simulink model "px4demo_attitude_system_GCS_combined_AttiGain3"  (R2016b)
settings: Solver=FixedStepDiscrete  StartTime=0.0  StopTime=inf  RelTol=1e-3
PostLoadFcn:
  | kFactor = 1.2;
  | 
  | KpRollAttitude = 0.630138625117681 / kFactor;
  | KiRollAttitude = 0.0552303199591522 / kFactor;
  | 
  | KpPitchAttitude = 0.630138625117681 / kFactor;
  | KiPitchAttitude = 0.0552303199591522 / kFactor;
  | 
  | KpRollRate = 1.31533836563383 / kFactor;
  | KiRollRate = 0.460338699849681 / kFactor;
  | 
  | KpPitchRate = 1.31533836563383 / kFactor;
  | KiPitchRate = 0.460338699849681 / kFactor;
  | 
  | KpYawRate = 1.31533836563383 / kFactor;
  | KiYawRate = 0.460338699849681 / kFactor;
undefined symbols (not defined in the file or in its folder): PX4_TUNE_ENUM, RGBLED_COLOR_ENUM, RGBLED_MODE_ENUM
libraries: pixhawk_slib_sensors_actuators x7, simulink x6, pixhawk_slib_ADC_serial x1
settings Model: Creator=Steve  LastModifiedBy=E6320
settings SolverCC: AutoInsertRateTranBlk=on
settings DataIOCC: LimitDataPoints=on  SaveFormat=Array
settings OptimizationCC: DefaultParameterBehavior=Inlined  LifeSpan=1  MaxStackSize=64
settings DebuggingCC: SolverPrmCheckMsg=warning  AllowSymbolicDim=off  SFUnexpectedBacktrackingDiag=warning  SFNoUnconditionalDefaultTransitionDiag=warning  SFExecutionAtInitializationDiag=none
settings HardwareCC: ProdBitPerPointer=32  ProdBitPerSizeT=32  ProdBitPerPtrDiffT=32  ProdLargestAtomicInteger=Long  ProdLargestAtomicFloat=Double  ProdWordSize=32  ProdHWDeviceType=ARM Compatible->ARM Cortex
settings ModelReferenceCC: PropagateSignalLabelsOutOfModel=off
settings RTWCC: SystemTargetFile=ert.tlc  HardwareBoard=Pixhawk PX4  TemplateMakefile=ert_default_tmf  Description=Embedded Coder  GenerateReport=on  Toolchain=Pixhawk Toolchain  IncludeHyperlinkInReport=on  LaunchReport=on  GenerateTraceReport=on  GenerateTraceReportSl=on  GenerateTraceReportSf=on  GenerateTraceReportEml=on  GenerateCodeMetricsReport=on
settings CodeAppCC: IgnoreCustomStorageClasses=off
settings ERTTargetCC: CodeReplacementLibrary=GCC ARM Cortex-A9  ExtModeTransport=1  ExtModeMexFile=ext_serial_win32_comm  ExtModeMexArgs=/dev/serial  ERTCustomFileTemplate=PX4_codertarget_file_process.tlc  ConvertIfToSwitch=off  SuppressUnreachableDefaultCases=off
settings ConfigComp: CovMetricSettings=dw  CovHtmlReporting=on  CovSaveCumulativeToWorkspaceVar=on  CovSaveSingleToWorkspaceVar=on  CovExternalEMLEnable=off  CovSFcnEnable=off

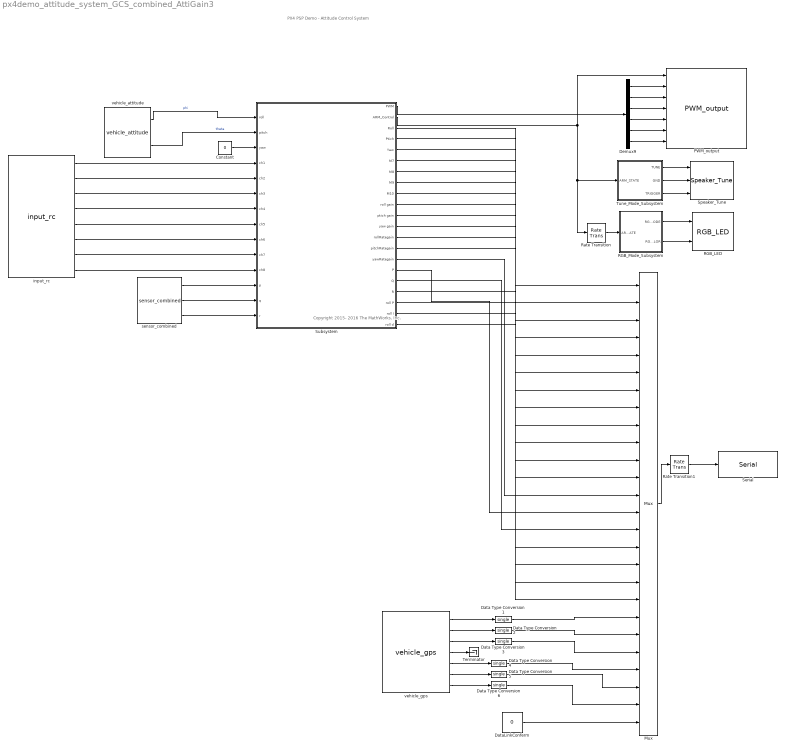
== system px4demo_attitude_system_GCS_combined_AttiGain3 ==
  note: PX4 PSP Demo - Attitude Control System
  note: Copyright 2015- 2016 The MathWorks, Inc.
  Constant : Constant  Value=0  OutDataTypeStr=single
  Data Type Conversion{1..6} (6 alike) : DataTypeConversion  OutDataTypeStr=single
  DataLinkConferm : Constant  Value=0  OutDataTypeStr=single
  Demux9 : Demux  Outputs=6
  Mux : Mux  Inputs=26
  PWM_output : pixhawk_slib_sensors_actuators/PWM_output  pwm_rate=250Hz  show_pwm1=on  show_pwm2=on  show_pwm3=on  show_pwm4=on  show_pwm5=on  show_pwm6=on  show_pwm7=off  show_pwm8=off
  RGB_LED : pixhawk_slib_sensors_actuators/RGB_LED
  RGB_Mode_Subsystem : Subsystem
  Rate Transition : RateTransition  OutPortSampleTime=1
  Rate Transition1 : RateTransition  OutPortSampleTime=1
  Serial : pixhawk_slib_ADC_serial/Serial  DeviceName=/dev/ttyS1  ReadOrWrite=Writing  BaudRateStr=57600  block=off  WriteStatus=on  Terminator=off  Header=off  NumBytesRead=4  TerminatorChar=\n  HeaderData=single('XD')  SimulateUsing=Code generation
  Speaker_Tune : pixhawk_slib_sensors_actuators/Speaker_Tune
  Subsystem : Subsystem
  Terminator : Terminator
  Tune_Mode_Subsystem : Subsystem
  input_rc : pixhawk_slib_sensors_actuators/input_rc  sampletime=1/250  channel1=on  channel2=on  channel3=on  channel4=on  channel5=on  channel6=on  channel7=on  channel8=on  ch_count=off  rssi=off  rc_failsafe=off  rc_lost=off  rc_inputsource=off
  sensor_combined : pixhawk_slib_sensors_actuators/sensor_combined  sampletime=1/250  show_mag=off  show_acc=off  show_gyro=on  show_baro=off  show_ts=off
  vehicle_attitude : pixhawk_slib_sensors_actuators/vehicle_attitude  sampletime=1/250  show_r=on  show_p=on  show_y=off  show_q=off
  vehicle_gps : pixhawk_slib_sensors_actuators/vehicle_gps  sampletime=1/250  show_ts_pos=off  show_alt=on  show_ts_gps=off  show_vel=on  show_fixtype=on  show_numsat=on
  wires:
  Demux9/6 -> PWM_output/7
  Demux9/5 -> PWM_output/6
  Demux9/4 -> PWM_output/5
  Demux9/2 -> PWM_output/3
  Demux9/3 -> PWM_output/4
  Demux9/1 -> PWM_output/2
  RGB_Mode_Subsystem/1(RGB_MODE) -> RGB_LED/1
  RGB_Mode_Subsystem/2(RGB_COLOR) -> RGB_LED/2
  Tune_Mode_Subsystem/1(TUNE) -> Speaker_Tune/1
  Tune_Mode_Subsystem/2(GND) -> Speaker_Tune/2
  Tune_Mode_Subsystem/3(TRIGGER) -> Speaker_Tune/3
  Subsystem/2(ARM_Control) -> PWM_output/1, Tune_Mode_Subsystem/1(ARM_STATE), Rate Transition/1
  vehicle_attitude/1 -> Subsystem/1(roll)  "phi"
  vehicle_attitude/2 -> Subsystem/2(pitch)  "theta"
  input_rc/1 -> Subsystem/4(ch1)
  input_rc/2 -> Subsystem/5(ch2)
  input_rc/3 -> Subsystem/6(ch3)
  input_rc/4 -> Subsystem/7(ch4)
  input_rc/5 -> Subsystem/8(ch5)
  Subsystem/1(PWM) -> Demux9/1
  Rate Transition/1 -> RGB_Mode_Subsystem/1(ARM_STATE)
  Mux/1 -> Rate Transition1/1
  Rate Transition1/1 -> Serial/1
  Subsystem/3(Roll) -> Mux/1
  Subsystem/4(Ptich) -> Mux/2
  Subsystem/5(Yaw) -> Mux/3
  Subsystem/6(M7) -> Mux/4
  Subsystem/7(M8) -> Mux/5
  Subsystem/8(M9) -> Mux/6
  Subsystem/9(M10) -> Mux/7
  Subsystem/10(roll gain) -> Mux/8
  Subsystem/11(ptich gain) -> Mux/9
  Subsystem/12(yaw gain) -> Mux/10
  Subsystem/13(rollRategain) -> Mux/11
  Subsystem/14(pitchRategain) -> Mux/12
  Subsystem/15(yawRategain) -> Mux/13
  sensor_combined/1 -> Subsystem/12(p)
  sensor_combined/2 -> Subsystem/13(q)
  sensor_combined/3 -> Subsystem/14(r)
  Constant/1 -> Subsystem/3(yaw)
  input_rc/6 -> Subsystem/9(ch6)
  input_rc/7 -> Subsystem/10(ch7)
  input_rc/8 -> Subsystem/11(ch8)
  vehicle_gps/2 -> Data Type Conversion2/1
  vehicle_gps/1 -> Data Type Conversion1/1
  vehicle_gps/3 -> Data Type Conversion3/1
  vehicle_gps/5 -> Data Type Conversion4/1
  vehicle_gps/6 -> Data Type Conversion5/1
  vehicle_gps/7 -> Data Type Conversion6/1
  vehicle_gps/4 -> Terminator/1
  Data Type Conversion1/1 -> Mux/20
  Data Type Conversion2/1 -> Mux/21
  Data Type Conversion3/1 -> Mux/22
  Data Type Conversion4/1 -> Mux/23
  Data Type Conversion5/1 -> Mux/24
  Data Type Conversion6/1 -> Mux/25
  DataLinkConferm/1 -> Mux/26
  Subsystem/18(R) -> Mux/16
  Subsystem/17(Q) -> Mux/15
  Subsystem/16(P) -> Mux/14
  Subsystem/19(roll P) -> Mux/17
  Subsystem/20(roll I) -> Mux/18
  Subsystem/21(roll d) -> Mux/19

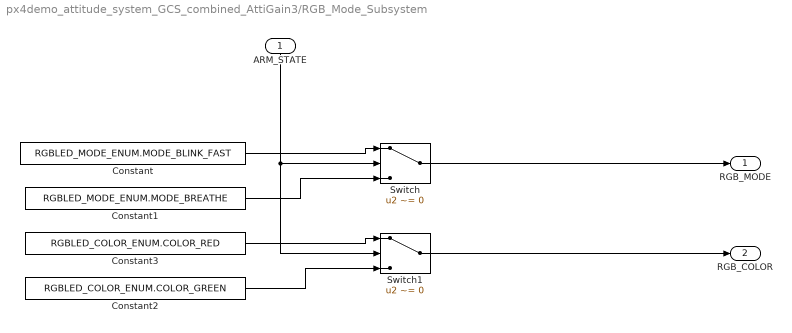
== system px4demo_attitude_system_GCS_combined_AttiGain3/RGB_Mode_Subsystem ==
  ARM_STATE : Inport
  Constant : Constant  Value=RGBLED_MODE_ENUM.MODE_BLINK_FAST  OutDataTypeStr=Enum: RGBLED_MODE_ENUM
  Constant1 : Constant  Value=RGBLED_MODE_ENUM.MODE_BREATHE  OutDataTypeStr=Enum: RGBLED_MODE_ENUM
  Constant2 : Constant  Value=RGBLED_COLOR_ENUM.COLOR_GREEN  OutDataTypeStr=Enum: RGBLED_COLOR_ENUM
  Constant3 : Constant  Value=RGBLED_COLOR_ENUM.COLOR_RED  OutDataTypeStr=Enum: RGBLED_COLOR_ENUM
  Switch : Switch  Criteria=u2 ~= 0  Threshold=1500  SampleTime=1/2
  Switch1 : Switch  Criteria=u2 ~= 0  Threshold=1500  SampleTime=1/2
  RGB_MODE : Outport
  RGB_COLOR : Outport  Port=2
  wires:
  ARM_STATE/1 -> Switch1/2, Switch/2
  Constant/1 -> Switch/1
  Constant1/1 -> Switch/3
  Switch/1 -> RGB_MODE/1
  Constant3/1 -> Switch1/1
  Constant2/1 -> Switch1/3
  Switch1/1 -> RGB_COLOR/1

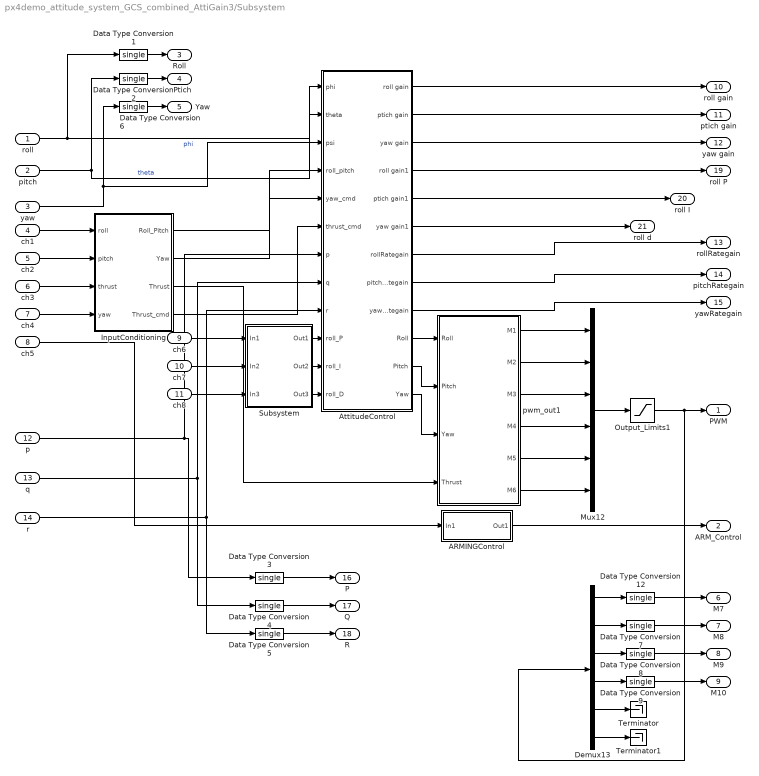
== system px4demo_attitude_system_GCS_combined_AttiGain3/Subsystem ==
  roll : Inport  OutDataTypeStr=single  PortDimensions=1
  pitch : Inport  Port=2  PortDimensions=1
  yaw : Inport  Port=3  PortDimensions=1
  ch1 : Inport  Port=4  OutDataTypeStr=uint16  PortDimensions=1
  ch2 : Inport  Port=5  OutDataTypeStr=uint16  PortDimensions=1
  ch3 : Inport  Port=6  OutDataTypeStr=uint16  PortDimensions=1
  ch4 : Inport  Port=7  OutDataTypeStr=uint16  PortDimensions=1
  ch5 : Inport  Port=8  OutDataTypeStr=uint16  PortDimensions=1  Interpolate=off
  ch6 : Inport  Port=9  OutDataTypeStr=uint16  PortDimensions=1
  ch7 : Inport  Port=10  OutDataTypeStr=uint16  PortDimensions=1
  ch8 : Inport  Port=11  OutDataTypeStr=uint16  PortDimensions=1
  p : Inport  Port=12  OutDataTypeStr=single  PortDimensions=1
  q : Inport  Port=13  OutDataTypeStr=single  PortDimensions=1
  r : Inport  Port=14  PortDimensions=1
  ARMINGControl : Subsystem
  AttitudeControl : Subsystem
  Data Type Conversion{1..9,12} (10 alike) : DataTypeConversion  OutDataTypeStr=single
  Demux13 : Demux  Outputs=6
  InputConditioning : Subsystem
  Mux12 : Mux  Inputs=6
  Output_Limits1 : Saturate  UpperLimit=2000  LowerLimit=1000
  Subsystem : Subsystem
  Terminator : Terminator
  Terminator1 : Terminator
  pwm_out1 : MATLAB Function  TreatAsAtomicUnit=on  SystemSampleTime=0.004
  PWM : Outport  PortDimensions=6
  ARM_Control : Outport  Port=2  PortDimensions=1
  Roll : Outport  Port=3  PortDimensions=1
  Ptich : Outport  Port=4  PortDimensions=1
  Yaw : Outport  Port=5  PortDimensions=1
  M7 : Outport  Port=6  PortDimensions=1
  M8 : Outport  Port=7  PortDimensions=1
  M9 : Outport  Port=8  PortDimensions=1
  M10 : Outport  Port=9  PortDimensions=1
  roll gain : Outport  Port=10
  ptich gain : Outport  Port=11
  yaw gain : Outport  Port=12
  rollRategain : Outport  Port=13
  pitchRategain : Outport  Port=14
  yawRategain : Outport  Port=15
  P : Outport  Port=16  PortDimensions=1
  Q : Outport  Port=17  PortDimensions=1
  R : Outport  Port=18  PortDimensions=1
  roll P : Outport  Port=19
  roll I : Outport  Port=20
  roll d : Outport  Port=21
  wires:
  Mux12/1 -> Output_Limits1/1
  InputConditioning/3(Thrust) -> pwm_out1/4(Thrust)
  roll/1 -> Data Type Conversion1/1, AttitudeControl/1(phi)  "phi"
  pitch/1 -> AttitudeControl/2(theta), Data Type Conversion2/1  "theta"
  InputConditioning/1(Roll_Pitch) -> AttitudeControl/4(roll_pitch)
  InputConditioning/2(Yaw) -> AttitudeControl/5(yaw_cmd)
  p/1 -> Data Type Conversion3/1, AttitudeControl/7(p)
  q/1 -> AttitudeControl/8(q), Data Type Conversion4/1
  r/1 -> AttitudeControl/9(r), Data Type Conversion5/1
  AttitudeControl/10(Roll) -> pwm_out1/1(Roll)
  AttitudeControl/11(Pitch) -> pwm_out1/2(Pitch)
  AttitudeControl/12(Yaw) -> pwm_out1/3(Yaw)
  ch5/1 -> ARMINGControl/1(In1)
  pwm_out1/1(M1) -> Mux12/1
  pwm_out1/2(M2) -> Mux12/2
  pwm_out1/3(M3) -> Mux12/3
  pwm_out1/4(M4) -> Mux12/4
  pwm_out1/5(M5) -> Mux12/5
  pwm_out1/6(M6) -> Mux12/6
  ch1/1 -> InputConditioning/1(roll)
  ch2/1 -> InputConditioning/2(pitch)
  ch4/1 -> InputConditioning/4(yaw)
  ch3/1 -> InputConditioning/3(thrust)
  ARMINGControl/1(Out1) -> ARM_Control/1
  InputConditioning/4(Thrust_cmd) -> AttitudeControl/6(thrust_cmd)
  Data Type Conversion1/1 -> Roll/1
  Data Type Conversion2/1 -> Ptich/1
  Output_Limits1/1 -> Demux13/1, PWM/1
  Data Type Conversion12/1 -> M7/1
  Data Type Conversion7/1 -> M8/1
  Data Type Conversion8/1 -> M9/1
  Data Type Conversion9/1 -> M10/1
  Demux13/1 -> Data Type Conversion12/1
  Demux13/2 -> Data Type Conversion7/1
  Demux13/3 -> Data Type Conversion8/1
  Demux13/4 -> Data Type Conversion9/1
  Demux13/5 -> Terminator/1
  AttitudeControl/1(roll gain) -> roll gain/1
  AttitudeControl/2(ptich gain) -> ptich gain/1
  AttitudeControl/7(rollRategain) -> rollRategain/1
  AttitudeControl/8(pitchRategain) -> pitchRategain/1
  Demux13/6 -> Terminator1/1
  Data Type Conversion3/1 -> P/1
  Data Type Conversion4/1 -> Q/1
  Data Type Conversion5/1 -> R/1
  AttitudeControl/9(yawRategain) -> yawRategain/1
  yaw/1 -> AttitudeControl/3(psi), Data Type Conversion6/1
  Data Type Conversion6/1 -> Yaw/1
  AttitudeControl/3(yaw gain) -> yaw gain/1
  AttitudeControl/6(yaw gain1) -> roll d/1
  AttitudeControl/5(ptich gain1) -> roll I/1
  AttitudeControl/4(roll gain1) -> roll P/1
  ch6/1 -> Subsystem/1(In1)
  ch7/1 -> Subsystem/2(In2)
  ch8/1 -> Subsystem/3(In3)
  Subsystem/1(Out1) -> AttitudeControl/10(roll_P)
  Subsystem/3(Out3) -> AttitudeControl/12(roll_D)
  Subsystem/2(Out2) -> AttitudeControl/11(roll_I)

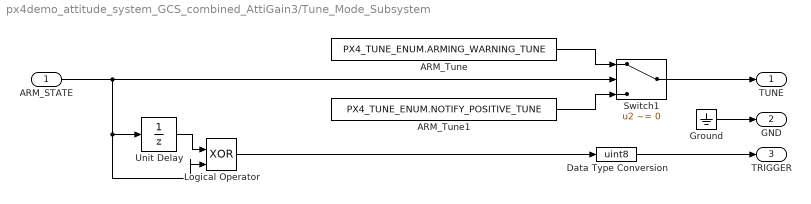
== system px4demo_attitude_system_GCS_combined_AttiGain3/Tune_Mode_Subsystem ==
  ARM_STATE : Inport
  ARM_Tune : Constant  Value=PX4_TUNE_ENUM.ARMING_WARNING_TUNE  OutDataTypeStr=Enum: PX4_TUNE_ENUM
  ARM_Tune1 : Constant  Value=PX4_TUNE_ENUM.NOTIFY_POSITIVE_TUNE  OutDataTypeStr=Enum: PX4_TUNE_ENUM
  Data Type Conversion : DataTypeConversion  OutDataTypeStr=uint8
  Ground : Ground
  Logical Operator : Logic  Operator=XOR  IconShape=distinctive  AllPortsSameDT=off  OutDataTypeStr=boolean
  Switch1 : Switch  Criteria=u2 ~= 0  Threshold=1500
  Unit Delay : UnitDelay  SampleTime=-1
  TUNE : Outport
  GND : Outport  Port=2
  TRIGGER : Outport  Port=3
  wires:
  Ground/1 -> GND/1
  Data Type Conversion/1 -> TRIGGER/1
  Switch1/1 -> TUNE/1
  ARM_Tune/1 -> Switch1/1
  ARM_Tune1/1 -> Switch1/3
  ARM_STATE/1 -> Logical Operator/2, Unit Delay/1, Switch1/2
  Unit Delay/1 -> Logical Operator/1
  Logical Operator/1 -> Data Type Conversion/1

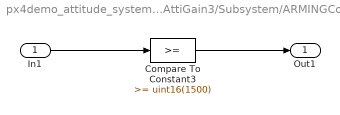
== system px4demo_attitude_system_GCS_combined_AttiGain3/Subsystem/ARMINGControl ==
  In1 : Inport
  Compare To Constant3 : simulink/Logic and Bit Operations/Compare To Constant  relop=>=  const=uint16(1500)  OutDataTypeStr=boolean
  Out1 : Outport
  wires:
  Compare To Constant3/1 -> Out1/1
  In1/1 -> Compare To Constant3/1

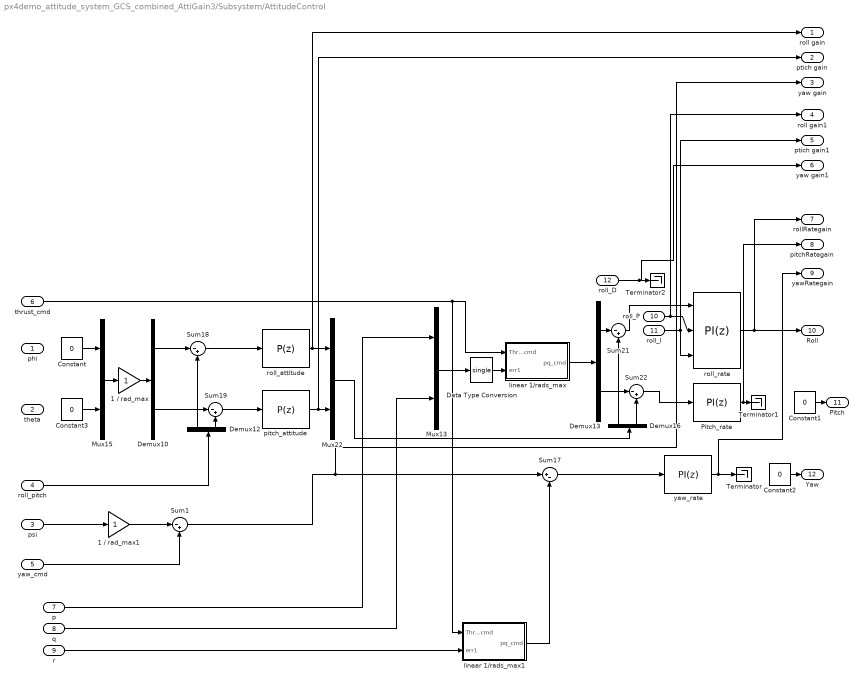
== system px4demo_attitude_system_GCS_combined_AttiGain3/Subsystem/AttitudeControl ==
  phi : Inport
  theta : Inport  Port=2
  psi : Inport  Port=3
  roll_pitch : Inport  Port=4
  yaw_cmd : Inport  Port=5
  thrust_cmd : Inport  Port=6
  p : Inport  Port=7
  q : Inport  Port=8
  r : Inport  Port=9
  roll_P : Inport  Port=10
  roll_I : Inport  Port=11
  roll_D : Inport  Port=12
  1 / rad_max : Gain
  1 / rad_max1 : Gain
  Constant{,1..3} (4 alike) : Constant  Value=0  OutDataTypeStr=single
  Data Type Conversion : DataTypeConversion  OutDataTypeStr=single
  Demux{10,12..13,16} (4 alike) : Demux  Outputs=2
  Mux13 : Mux  Inputs=2
  Mux15 : Mux  Inputs=2
  Mux22 : Mux  Inputs=2
  Pitch_rate : simulink/Continuous/PID Controller  Controller=PI  TimeDomain=Discrete-time  SampleTime=-1  IntegratorMethod=Forward Euler  FilterMethod=Forward Euler  Form=Parallel  UseFilter=on  ControllerParametersSource=internal  P=5  I=0.01  D=0.0024  N=100  InitialConditionSource=internal  InitialConditionForIntegrator=0  InitialConditionForFilter=0  ExternalReset=none  LimitOutput=on  UpperSaturationLimit=1  LowerSaturationLimit=-1  LinearizeAsGain=on  AntiWindupMode=clamping  Kb=1  TrackingMode=off  Kt=1  PParamMin=[]  PParamMax=[]  IParamMin=[]  IParamMax=[]  DParamMin=[]  DParamMax=[]  NParamMin=[]  NParamMax=[]  KbParamMin=[]  KbParamMax=[]  KtParamMin=[]  KtParamMax=[]  POutMin=[]  POutMax=[]  IOutMin=[]  IOutMax=[]  DOutMin=[]  DOutMax=[]  NOutMin=[]  NOutMax=[]  KbOutMin=[]  KbOutMax=[]  KtOutMin=[]  KtOutMax=[]  IntegratorOutMin=[]  IntegratorOutMax=[]  FilterOutMin=[]  FilterOutMax=[]  SumOutMin=[]  SumOutMax=[]  SumI1OutMin=[]  SumI1OutMax=[]  SumI2OutMin=[]  SumI2OutMax=[]  SumI3OutMin=[]  SumI3OutMax=[]  SumDOutMin=[]  SumDOutMax=[]  SaturationOutMin=[]  SaturationOutMax=[]  IntegratorContinuousStateAttributes=''  IntegratorStateMustResolveToSignalObject=off  IntegratorRTWStateStorageClass=Auto  FilterContinuousStateAttributes=''  FilterStateMustResolveToSignalObject=off  FilterRTWStateStorageClass=Auto  DifferentiatorICPrevScaledInput=0  DifferentiatorOutMin=[]  DifferentiatorOutMax=[]
  Sum{1,18..19,21..22} (5 alike) : Sum  Inputs=|-+
  Sum17 : Sum  Inputs=|+-
  Terminator : Terminator
  Terminator1 : Terminator
  Terminator2 : Terminator
  linear 1/rads_max : MATLAB Function  TreatAsAtomicUnit=on
  linear 1/rads_max1 : MATLAB Function  TreatAsAtomicUnit=on
  pitch_attitude : simulink/Continuous/PID Controller  Controller=P  TimeDomain=Discrete-time  SampleTime=-1  IntegratorMethod=Forward Euler  FilterMethod=Forward Euler  Form=Parallel  UseFilter=on  ControllerParametersSource=internal  P=1  I=0.05  D=0.01  N=100  InitialConditionSource=internal  InitialConditionForIntegrator=0  InitialConditionForFilter=0  ExternalReset=none  LimitOutput=on  UpperSaturationLimit=1  LowerSaturationLimit=-1  LinearizeAsGain=on  AntiWindupMode=clamping  Kb=1  TrackingMode=off  Kt=1  PParamMin=[]  PParamMax=[]  IParamMin=[]  IParamMax=[]  DParamMin=[]  DParamMax=[]  NParamMin=[]  NParamMax=[]  KbParamMin=[]  KbParamMax=[]  KtParamMin=[]  KtParamMax=[]  POutMin=[]  POutMax=[]  IOutMin=[]  IOutMax=[]  DOutMin=[]  DOutMax=[]  NOutMin=[]  NOutMax=[]  KbOutMin=[]  KbOutMax=[]  KtOutMin=[]  KtOutMax=[]  IntegratorOutMin=[]  IntegratorOutMax=[]  FilterOutMin=[]  FilterOutMax=[]  SumOutMin=[]  SumOutMax=[]  SumI1OutMin=[]  SumI1OutMax=[]  SumI2OutMin=[]  SumI2OutMax=[]  SumI3OutMin=[]  SumI3OutMax=[]  SumDOutMin=[]  SumDOutMax=[]  SaturationOutMin=[]  SaturationOutMax=[]  IntegratorContinuousStateAttributes=''  IntegratorStateMustResolveToSignalObject=off  IntegratorRTWStateStorageClass=Auto  FilterContinuousStateAttributes=''  FilterStateMustResolveToSignalObject=off  FilterRTWStateStorageClass=Auto  DifferentiatorICPrevScaledInput=0  DifferentiatorOutMin=[]  DifferentiatorOutMax=[]
  roll_attitude : simulink/Continuous/PID Controller  Controller=P  TimeDomain=Discrete-time  SampleTime=-1  IntegratorMethod=Forward Euler  FilterMethod=Forward Euler  Form=Parallel  UseFilter=on  ControllerParametersSource=internal  P=1  I=0.04  D=0.01  N=100  InitialConditionSource=internal  InitialConditionForIntegrator=0  InitialConditionForFilter=0  ExternalReset=none  LimitOutput=on  UpperSaturationLimit=1  LowerSaturationLimit=-1  LinearizeAsGain=on  AntiWindupMode=clamping  Kb=1  TrackingMode=off  Kt=1  PParamMin=[]  PParamMax=[]  IParamMin=[]  IParamMax=[]  DParamMin=[]  DParamMax=[]  NParamMin=[]  NParamMax=[]  KbParamMin=[]  KbParamMax=[]  KtParamMin=[]  KtParamMax=[]  POutMin=[]  POutMax=[]  IOutMin=[]  IOutMax=[]  DOutMin=[]  DOutMax=[]  NOutMin=[]  NOutMax=[]  KbOutMin=[]  KbOutMax=[]  KtOutMin=[]  KtOutMax=[]  IntegratorOutMin=[]  IntegratorOutMax=[]  FilterOutMin=[]  FilterOutMax=[]  SumOutMin=[]  SumOutMax=[]  SumI1OutMin=[]  SumI1OutMax=[]  SumI2OutMin=[]  SumI2OutMax=[]  SumI3OutMin=[]  SumI3OutMax=[]  SumDOutMin=[]  SumDOutMax=[]  SaturationOutMin=[]  SaturationOutMax=[]  IntegratorContinuousStateAttributes=''  IntegratorStateMustResolveToSignalObject=off  IntegratorRTWStateStorageClass=Auto  FilterContinuousStateAttributes=''  FilterStateMustResolveToSignalObject=off  FilterRTWStateStorageClass=Auto  DifferentiatorICPrevScaledInput=0  DifferentiatorOutMin=[]  DifferentiatorOutMax=[]
  roll_rate : simulink/Continuous/PID Controller  Controller=PI  TimeDomain=Discrete-time  SampleTime=-1  IntegratorMethod=Forward Euler  FilterMethod=Forward Euler  Form=Parallel  UseFilter=on  ControllerParametersSource=external  P=5  I=0.01  D=0.015  N=100  InitialConditionSource=internal  InitialConditionForIntegrator=0  InitialConditionForFilter=0  ExternalReset=none  LimitOutput=on  UpperSaturationLimit=1  LowerSaturationLimit=-1  LinearizeAsGain=on  AntiWindupMode=clamping  Kb=1  TrackingMode=off  Kt=1  PParamMin=[]  PParamMax=[]  IParamMin=[]  IParamMax=[]  DParamMin=[]  DParamMax=[]  NParamMin=[]  NParamMax=[]  KbParamMin=[]  KbParamMax=[]  KtParamMin=[]  KtParamMax=[]  POutMin=[]  POutMax=[]  IOutMin=[]  IOutMax=[]  DOutMin=[]  DOutMax=[]  NOutMin=[]  NOutMax=[]  KbOutMin=[]  KbOutMax=[]  KtOutMin=[]  KtOutMax=[]  IntegratorOutMin=[]  IntegratorOutMax=[]  FilterOutMin=[]  FilterOutMax=[]  SumOutMin=[]  SumOutMax=[]  SumI1OutMin=[]  SumI1OutMax=[]  SumI2OutMin=[]  SumI2OutMax=[]  SumI3OutMin=[]  SumI3OutMax=[]  SumDOutMin=[]  SumDOutMax=[]  SaturationOutMin=[]  SaturationOutMax=[]  IntegratorContinuousStateAttributes=''  IntegratorStateMustResolveToSignalObject=off  IntegratorRTWStateStorageClass=Auto  FilterContinuousStateAttributes=''  FilterStateMustResolveToSignalObject=off  FilterRTWStateStorageClass=Auto  DifferentiatorICPrevScaledInput=0  DifferentiatorOutMin=[]  DifferentiatorOutMax=[]
  yaw_rate : simulink/Continuous/PID Controller  Controller=PI  TimeDomain=Discrete-time  SampleTime=-1  IntegratorMethod=Forward Euler  FilterMethod=Forward Euler  Form=Parallel  UseFilter=on  ControllerParametersSource=internal  P=0.87  I=0.3  D=0  N=100  InitialConditionSource=internal  InitialConditionForIntegrator=0  InitialConditionForFilter=0  ExternalReset=none  LimitOutput=on  UpperSaturationLimit=1  LowerSaturationLimit=-1  LinearizeAsGain=on  AntiWindupMode=back-calculation  Kb=1  TrackingMode=off  Kt=1  PParamMin=[]  PParamMax=[]  IParamMin=[]  IParamMax=[]  DParamMin=[]  DParamMax=[]  NParamMin=[]  NParamMax=[]  KbParamMin=[]  KbParamMax=[]  KtParamMin=[]  KtParamMax=[]  POutMin=[]  POutMax=[]  IOutMin=[]  IOutMax=[]  DOutMin=[]  DOutMax=[]  NOutMin=[]  NOutMax=[]  KbOutMin=[]  KbOutMax=[]  KtOutMin=[]  KtOutMax=[]  IntegratorOutMin=[]  IntegratorOutMax=[]  FilterOutMin=[]  FilterOutMax=[]  SumOutMin=[]  SumOutMax=[]  SumI1OutMin=[]  SumI1OutMax=[]  SumI2OutMin=[]  SumI2OutMax=[]  SumI3OutMin=[]  SumI3OutMax=[]  SumDOutMin=[]  SumDOutMax=[]  SaturationOutMin=[]  SaturationOutMax=[]  IntegratorContinuousStateAttributes=''  IntegratorStateMustResolveToSignalObject=off  IntegratorRTWStateStorageClass=Auto  FilterContinuousStateAttributes=''  FilterStateMustResolveToSignalObject=off  FilterRTWStateStorageClass=Auto  DifferentiatorICPrevScaledInput=0  DifferentiatorOutMin=[]  DifferentiatorOutMax=[]
  roll gain : Outport
  ptich gain : Outport  Port=2
  yaw gain : Outport  Port=3
  roll gain1 : Outport  Port=4
  ptich gain1 : Outport  Port=5
  yaw gain1 : Outport  Port=6
  rollRategain : Outport  Port=7
  pitchRategain : Outport  Port=8
  yawRategain : Outport  Port=9
  Roll : Outport  Port=10
  Pitch : Outport  Port=11
  Yaw : Outport  Port=12
  wires:
  Mux22/1 -> Demux16/1
  Mux15/1 -> 1 / rad_max/1
  roll_rate/1 -> rollRategain/1, Roll/1
  Sum19/1 -> pitch_attitude/1
  pitch_attitude/1 -> Mux22/2, ptich gain/1
  Demux16/1 -> Sum21/2
  roll_pitch/1 -> Demux12/1
  Demux16/2 -> Sum22/2
  Demux12/1 -> Sum18/2
  Demux12/2 -> Sum19/2
  Demux10/1 -> Sum18/1
  Demux10/2 -> Sum19/1
  1 / rad_max/1 -> Demux10/1
  Sum18/1 -> roll_attitude/1
  Sum22/1 -> Pitch_rate/1
  Sum17/1 -> yaw_rate/1
  Demux13/1 -> Sum21/1
  Demux13/2 -> Sum22/1
  Sum21/1 -> roll_rate/1
  Data Type Conversion/1 -> linear 1/rads_max/2(err1)
  Mux13/1 -> Data Type Conversion/1
  linear 1/rads_max/1(pq_cmd) -> Demux13/1
  thrust_cmd/1 -> linear 1/rads_max1/1(Thrust_cmd), linear 1/rads_max/1(Thrust_cmd)
  roll_attitude/1 -> roll gain/1, Mux22/1
  psi/1 -> 1 / rad_max1/1
  1 / rad_max1/1 -> Sum1/1
  yaw_cmd/1 -> Sum1/2
  linear 1/rads_max1/1(pq_cmd) -> Sum17/2
  Sum1/1 -> yaw gain/1, Sum17/1
  p/1 -> Mux13/1
  q/1 -> Mux13/2
  r/1 -> linear 1/rads_max1/2(err1)
  roll_P/1 -> roll gain1/1, roll_rate/2
  roll_I/1 -> ptich gain1/1, roll_rate/3
  roll_D/1 -> yaw gain1/1, Terminator2/1
  yaw_rate/1 -> Terminator/1, yawRategain/1
  Constant1/1 -> Pitch/1
  Pitch_rate/1 -> pitchRategain/1, Terminator1/1
  Constant2/1 -> Yaw/1
  Constant/1 -> Mux15/1
  Constant3/1 -> Mux15/2

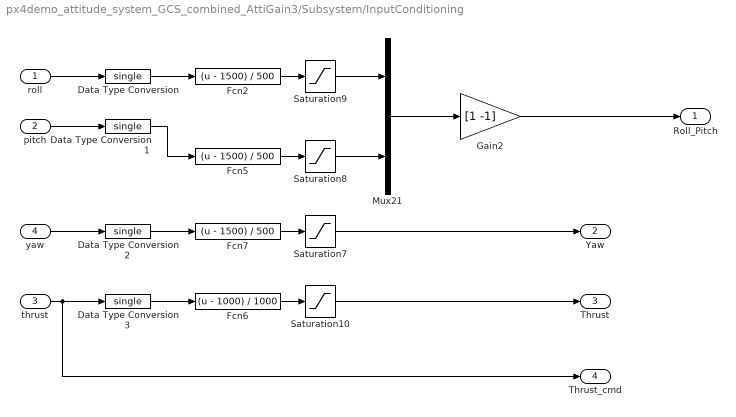
== system px4demo_attitude_system_GCS_combined_AttiGain3/Subsystem/InputConditioning ==
  roll : Inport
  pitch : Inport  Port=2
  thrust : Inport  Port=3
  yaw : Inport  Port=4
  Data Type Conversion{,1..3} (4 alike) : DataTypeConversion  OutDataTypeStr=single
  Fcn2 : Fcn  Expr=(u - 1500) / 500
  Fcn5 : Fcn  Expr=(u - 1500) / 500
  Fcn6 : Fcn  Expr=(u - 1000) / 1000
  Fcn7 : Fcn  Expr=(u - 1500) / 500
  Gain2 : Gain  Gain=[1 -1]  OutDataTypeStr=Inherit: Inherit via back propagation
  Mux21 : Mux  Inputs=2
  Saturation10 : Saturate  UpperLimit=1  LowerLimit=0
  Saturation7 : Saturate  UpperLimit=1  LowerLimit=-1
  Saturation8 : Saturate  UpperLimit=1  LowerLimit=-1
  Saturation9 : Saturate  UpperLimit=1  LowerLimit=-1
  Roll_Pitch : Outport
  Yaw : Outport  Port=2
  Thrust : Outport  Port=3
  Thrust_cmd : Outport  Port=4
  wires:
  Saturation10/1 -> Thrust/1
  Saturation7/1 -> Yaw/1
  Gain2/1 -> Roll_Pitch/1
  Mux21/1 -> Gain2/1
  Saturation8/1 -> Mux21/2
  Fcn6/1 -> Saturation10/1
  thrust/1 -> Thrust_cmd/1, Data Type Conversion3/1
  Fcn2/1 -> Saturation9/1
  Fcn5/1 -> Saturation8/1
  Saturation9/1 -> Mux21/1
  Fcn7/1 -> Saturation7/1
  yaw/1 -> Data Type Conversion2/1
  pitch/1 -> Data Type Conversion1/1
  roll/1 -> Data Type Conversion/1
  Data Type Conversion/1 -> Fcn2/1
  Data Type Conversion1/1 -> Fcn5/1
  Data Type Conversion2/1 -> Fcn7/1
  Data Type Conversion3/1 -> Fcn6/1

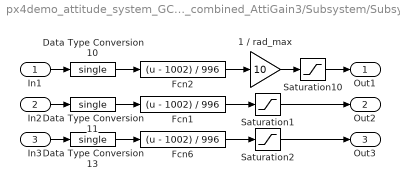
== system px4demo_attitude_system_GCS_combined_AttiGain3/Subsystem/Subsystem ==
  In1 : Inport
  In2 : Inport  Port=2
  In3 : Inport  Port=3
  1 / rad_max : Gain  Gain=10
  Data Type Conversion10 : DataTypeConversion  OutDataTypeStr=single
  Data Type Conversion11 : DataTypeConversion  OutDataTypeStr=single
  Data Type Conversion13 : DataTypeConversion  OutDataTypeStr=single
  Fcn1 : Fcn  Expr=(u - 1002) / 996
  Fcn2 : Fcn  Expr=(u - 1002) / 996
  Fcn6 : Fcn  Expr=(u - 1002) / 996
  Saturation1 : Saturate  UpperLimit=1  LowerLimit=0
  Saturation10 : Saturate  UpperLimit=3  LowerLimit=0
  Saturation2 : Saturate  UpperLimit=1  LowerLimit=0
  Out1 : Outport
  Out2 : Outport  Port=2
  Out3 : Outport  Port=3
  wires:
  Data Type Conversion13/1 -> Fcn6/1
  Fcn6/1 -> Saturation2/1
  Fcn2/1 -> 1 / rad_max/1
  Data Type Conversion11/1 -> Fcn1/1
  In3/1 -> Data Type Conversion13/1
  Data Type Conversion10/1 -> Fcn2/1
  In2/1 -> Data Type Conversion11/1
  In1/1 -> Data Type Conversion10/1
  Fcn1/1 -> Saturation1/1
  Saturation10/1 -> Out1/1
  Saturation1/1 -> Out2/1
  Saturation2/1 -> Out3/1
  1 / rad_max/1 -> Saturation10/1

== matlab function px4demo_attitude_system_GCS_combined_AttiGain3/Subsystem/AttitudeControl/linear 1//rads_max1 ==
  data: Thrust_cmd input; pq_cmd output; err1 input
function pq_cmd  = fcn(Thrust_cmd,err1)

% T = 1225. rads max = 3
% T = 1400. rads max = 20

T1 = 1225; T2 = 1400;
p1 = 4; p2 = 25;
m = (p2-p1)/(T2-T1);
b = p1 - m*T1;

y = single(max(4,m*min(1946,max(1135,Thrust_cmd)) + b));

pq_cmd = single(err1/y);

== matlab function px4demo_attitude_system_GCS_combined_AttiGain3/Subsystem/AttitudeControl/linear 1//rads_max ==
  data: Thrust_cmd input; pq_cmd output; err1 input
function pq_cmd  = fcn(Thrust_cmd,err1)

% T = 1225. rads max = 3
% T = 1400. rads max = 20

T1 = 1225; T2 = 1400;
p1 = 3; p2 = 12;
m = (p2-p1)/(T2-T1);
b = p1 - m*T1;

y = single(max(3,m*min(1946,max(1135,Thrust_cmd)) + b));

pq_cmd = single(err1/y);

== matlab function px4demo_attitude_system_GCS_combined_AttiGain3/Subsystem/pwm_out1 ==
  data: Roll input; M1 output; Pitch input; Yaw input; Thrust input; M2 output; M3 output; M4 output; M5 output; M6 output
function [M1, M2, M3, M4, M5, M6] = motor_mixer(Roll, Pitch, Yaw, Thrust)

idle_PWM = uint16(1145);

% Quad X
M1 = uint16(single(((Roll + Pitch - Yaw) / 2 * Thrust + Thrust) * single(1000))) + idle_PWM;
M2 = uint16(single(((-Roll + Pitch + Yaw) / 2 * Thrust + Thrust) * single(1000))) + idle_PWM;
M3 = uint16(single(((-Roll - Pitch - Yaw) / 2 * Thrust + Thrust) * single(1000))) + idle_PWM;
M4 = uint16(single(((Roll - Pitch + Yaw) / 2 * Thrust + Thrust) * single(1000))) + idle_PWM;
M5 = uint16(1000);
M6 = uint16(1000);
% M1 = uint16(single(((Roll + Pitch - Yaw)  + Thrust) * single(1000))) + idle_PWM;
% M2 = uint16(single(((-Roll + Pitch + Yaw)  + Thrust) * single(1000))) + idle_PWM;
% M3 = uint16(single(((-Roll - Pitch - Yaw)  + Thrust) * single(1000))) + idle_PWM;
% M4 = uint16(single(((Roll - Pitch + Yaw)  + Thrust) * single(1000))) + idle_PWM;
% M5 = uint16(1000);
% M6 = uint16(1000);

% Quad +
% M1 = ((Pitch - Yaw) * Thrust / 2 + Thrust) * 1000 + idle_PWM;
% M2 = ((-Roll + Yaw) * Thrust / 2 + Thrust) * 1000 + idle_PWM;
% M3 = ((-Pitch - Yaw) * Thrust / 2 + Thrust) * 1000 + idle_PWM;
% M4 = ((Roll + Yaw) * Thrust / 2 + Thrust) * 1000 + idle_PWM;
% M5 = 1000;
% M6 = 1000;
% M7 = 1000;
% M8 = 1000;

% Hex X
% M1 = ((Pitch + Roll / 2 - Yaw) * Thrust / 2 + Thrust) * 1000 + idle_PWM;
% M2 = ((Pitch - Roll / 2 + Yaw) * Thrust / 2 + Thrust) * 1000 + idle_PWM;
% M3 = ((-Roll - Yaw) * Thrust / 2 + Thrust) * 1000 + idle_PWM;
% M4 = ((-Pitch - Roll / 2 + Yaw) * Thrust / 2 + Thrust) * 1000 + idle_PWM;
% M5 = ((-Pitch + Roll / 2 - Yaw) * Thrust / 2 + Thrust) * 1000 + idle_PWM;
% M6 = ((Roll + Yaw) * Thrust / 2 + Thrust) * 1000 + idle_PWM;
% M7 = 1000;
% M8 = 1000;

% Hex X (From Adam)
% M1 = uint16(single(((-Roll - Yaw) * Thrust / 3 + Thrust) * single(1000))) + idle_PWM;
% M2 = uint16(single(((Roll + Yaw) * Thrust / 3 + Thrust) * single(1000))) + idle_PWM;
% M3 = uint16(single(((Pitch + (Roll / 2) - Yaw) * Thrust / 3 + Thrust) * single(1000))) + idle_PWM;
% M4 = uint16(single(((-Pitch - (Roll / 2) + Yaw) * Thrust / 3 + Thrust) * single(1000))) + idle_PWM;
% M5 = uint16(single(((Pitch - (Roll / 2) + Yaw) * Thrust / 3 + Thrust) * single(1000))) + idle_PWM;
% M6 = uint16(single(((-Pitch + (Roll / 2) - Yaw) * Thrust / 3 + Thrust) * single(1000))) + idle_PWM;

% Hex X (Version 2)
% Roll/Yaw
% M1 = ((-Roll - Yaw) * Thrust / 2 + Thrust) * 1000 + idle_PWM;
% M2 = ((Roll + Yaw) * Thrust / 2 + Thrust) * 1000 + idle_PWM;
% % + Pitch/Roll
% M6 = ((Pitch + Roll / 2 - Yaw) * Thrust / 2 + Thrust) * 1000 + idle_PWM;
% M4 = ((Pitch - Roll / 2 + Yaw) * Thrust / 2 + Thrust) * 1000 + idle_PWM;
% % - Pitch/Roll
% M5 = ((-Pitch - Roll / 2 + Yaw) * Thrust / 2 + Thrust) * 1000 + idle_PWM;
% M3 = ((-Pitch + Roll / 2 - Yaw) * Thrust / 2 + Thrust) * 1000 + idle_PWM;
